simulink model "TopLevelSim"  (R2024b)
settings: Solver=FixedStepDiscrete  StartTime=0.0  StopTime=sysParams.FPGAClkPeriod*1e4  RelTol=1e-3
PreLoadFcn:
  | init;
undefined symbols (not defined in the file): bfCoeffs_fxp, chanConfig, const_16APSK, const_64APSK, FXP, iChain, modEnable, modSel, OFDMmodType, SC, SCmodType, sysParams, tuningWord, txData
libraries: hdlsllib x20, commdigbbndpm3 x8, commdigbbndam3 x8, dspmlti4 x8, dsphdlfiltering2 x8, whdlmod x4, dsphdlsigops2 x4
(part 2 of 2)

== system TopLevelSim/Top Level/Baseband Signal Generator/channel1/Baseband Modulator/OFDM Modulator/mapper ==
  txBits : Inport
  OFDMmodType : Inport  Port=2
  16-APSK : LookupNDDirect  NumberOfTableDimensions=1  Table=const_16APSK  DiagnosticForOutOfRangeInput=Error
  64-APSK : LookupNDDirect  NumberOfTableDimensions=1  Table=const_64APSK  DiagnosticForOutOfRangeInput=Error
  Bit Slice : hdlsllib/Logic and Bit Operations/Bit Slice  lidx=3  ridx=0
  Bit Slice1 : hdlsllib/Logic and Bit Operations/Bit Slice  lidx=1  ridx=0
  Multiport Switch : MultiPortSwitch  DataPortOrder=Zero-based contiguous  Inputs=4  zeroidx=on  OutDataTypeStr=fixdt(1,FXP.sampWL,FXP.sampFL)  SaturateOnIntegerOverflow=off
  QPSK Modulator Baseband : commdigbbndpm3/QPSK Modulator Baseband  InType=Integer  Enc=Gray  Ph=pi/4  outDtype=Fixed-point  outWordLen=FXP.sampWL  outUDDataType=sfix(16)  outFracLenMode=User-defined  outFracLen=FXP.sampFL  outDataTypeStr=fixdt(1,FXP.sampWL,FXP.sampFL)  outLastDataTypeStr=fixdt(1,FXP.sampWL,FXP.sampFL)
  Rectangular QAM Modulator Baseband : commdigbbndam3/Rectangular QAM Modulator Baseband  M=16  InType=Integer  Enc=Gray  Mapping=[0:15]  PowType=Average Power  MinDist=2  AvgPow=1  PeakPow=1  Ph=0  outDtype=Fixed-point  outWordLen=FXP.sampWL  outUDDataType=sfix(16)  outFracLenMode=User-defined  outFracLen=FXP.sampFL  outDataTypeStr=fixdt(1,FXP.sampWL,FXP.sampFL)  outLastDataTypeStr=fixdt(1,FXP.sampWL,FXP.sampFL)
  tx_IQ : Outport  VectorParamsAs1DForOutWhenUnconnected=off
  wires:
  Bit Slice1/1 -> QPSK Modulator Baseband/1
  Bit Slice/1 -> 16-APSK/1, Rectangular QAM Modulator Baseband/1
  txBits/1 -> Bit Slice1/1, Bit Slice/1, 64-APSK/1
  Multiport Switch/1 -> tx_IQ/1
  64-APSK/1 -> Multiport Switch/5
  16-APSK/1 -> Multiport Switch/4
  Rectangular QAM Modulator Baseband/1 -> Multiport Switch/3
  QPSK Modulator Baseband/1 -> Multiport Switch/2
  OFDMmodType/1 -> Multiport Switch/1

== system TopLevelSim/Top Level/Baseband Signal Generator/channel1/Baseband Modulator/SC Modulator/mapper ==
  txBits : Inport
  SCmodType : Inport  Port=2
  16-APSK : LookupNDDirect  NumberOfTableDimensions=1  Table=const_16APSK  DiagnosticForOutOfRangeInput=Error  TableDataTypeStr=fixdt(1,FXP.sampWL,FXP.sampFL)
  Bit Slice : hdlsllib/Logic and Bit Operations/Bit Slice  lidx=3  ridx=0
  Bit Slice1 : hdlsllib/Logic and Bit Operations/Bit Slice  lidx=1  ridx=0
  Multiport Switch : MultiPortSwitch  DataPortOrder=Zero-based contiguous  zeroidx=on  OutDataTypeStr=fixdt(1,FXP.sampWL,FXP.sampFL)  SaturateOnIntegerOverflow=off  InputSameDT=off
  QPSK Modulator Baseband : commdigbbndpm3/QPSK Modulator Baseband  InType=Integer  Enc=Gray  Ph=pi/4  outDtype=Fixed-point  outWordLen=FXP.sampWL  outUDDataType=sfix(16)  outFracLenMode=User-defined  outFracLen=FXP.sampFL  outDataTypeStr=fixdt(1,FXP.sampWL,FXP.sampFL)  outLastDataTypeStr=fixdt(1,FXP.sampWL,FXP.sampFL)
  Rectangular QAM Modulator Baseband : commdigbbndam3/Rectangular QAM Modulator Baseband  M=16  InType=Integer  Enc=Gray  Mapping=[0:15]  PowType=Average Power  MinDist=2  AvgPow=1  PeakPow=1  Ph=0  outDtype=Fixed-point  outWordLen=FXP.sampWL  outUDDataType=sfix(16)  outFracLenMode=User-defined  outFracLen=FXP.sampFL  outDataTypeStr=fixdt(1,FXP.sampWL,FXP.sampFL)  outLastDataTypeStr=fixdt(1,FXP.sampWL,FXP.sampFL)
  tx_IQ : Outport
  wires:
  Bit Slice1/1 -> QPSK Modulator Baseband/1
  Bit Slice/1 -> 16-APSK/1, Rectangular QAM Modulator Baseband/1
  txBits/1 -> Bit Slice1/1, Bit Slice/1
  QPSK Modulator Baseband/1 -> Multiport Switch/2
  Rectangular QAM Modulator Baseband/1 -> Multiport Switch/4
  SCmodType/1 -> Multiport Switch/1
  Multiport Switch/1 -> tx_IQ/1
  16-APSK/1 -> Multiport Switch/3

== system TopLevelSim/Top Level/Baseband Signal Generator/channel2/Baseband Modulator/OFDM Modulator/mapper ==
  txBits : Inport
  OFDMmodType : Inport  Port=2
  16-APSK : LookupNDDirect  NumberOfTableDimensions=1  Table=const_16APSK  DiagnosticForOutOfRangeInput=Error
  64-APSK : LookupNDDirect  NumberOfTableDimensions=1  Table=const_64APSK  DiagnosticForOutOfRangeInput=Error
  Bit Slice : hdlsllib/Logic and Bit Operations/Bit Slice  lidx=3  ridx=0
  Bit Slice1 : hdlsllib/Logic and Bit Operations/Bit Slice  lidx=1  ridx=0
  Multiport Switch : MultiPortSwitch  DataPortOrder=Zero-based contiguous  Inputs=4  zeroidx=on  OutDataTypeStr=fixdt(1,FXP.sampWL,FXP.sampFL)  SaturateOnIntegerOverflow=off
  QPSK Modulator Baseband : commdigbbndpm3/QPSK Modulator Baseband  InType=Integer  Enc=Gray  Ph=pi/4  outDtype=Fixed-point  outWordLen=FXP.sampWL  outUDDataType=sfix(16)  outFracLenMode=User-defined  outFracLen=FXP.sampFL  outDataTypeStr=fixdt(1,FXP.sampWL,FXP.sampFL)  outLastDataTypeStr=fixdt(1,FXP.sampWL,FXP.sampFL)
  Rectangular QAM Modulator Baseband : commdigbbndam3/Rectangular QAM Modulator Baseband  M=16  InType=Integer  Enc=Gray  Mapping=[0:15]  PowType=Average Power  MinDist=2  AvgPow=1  PeakPow=1  Ph=0  outDtype=Fixed-point  outWordLen=FXP.sampWL  outUDDataType=sfix(16)  outFracLenMode=User-defined  outFracLen=FXP.sampFL  outDataTypeStr=fixdt(1,FXP.sampWL,FXP.sampFL)  outLastDataTypeStr=fixdt(1,FXP.sampWL,FXP.sampFL)
  tx_IQ : Outport  VectorParamsAs1DForOutWhenUnconnected=off
  wires:
  OFDMmodType/1 -> Multiport Switch/1
  QPSK Modulator Baseband/1 -> Multiport Switch/2
  Rectangular QAM Modulator Baseband/1 -> Multiport Switch/3
  16-APSK/1 -> Multiport Switch/4
  64-APSK/1 -> Multiport Switch/5
  Multiport Switch/1 -> tx_IQ/1
  txBits/1 -> 64-APSK/1, Bit Slice/1, Bit Slice1/1
  Bit Slice/1 -> Rectangular QAM Modulator Baseband/1, 16-APSK/1
  Bit Slice1/1 -> QPSK Modulator Baseband/1

== system TopLevelSim/Top Level/Baseband Signal Generator/channel2/Baseband Modulator/SC Modulator/mapper ==
  txBits : Inport
  SCmodType : Inport  Port=2
  16-APSK : LookupNDDirect  NumberOfTableDimensions=1  Table=const_16APSK  DiagnosticForOutOfRangeInput=Error  TableDataTypeStr=fixdt(1,FXP.sampWL,FXP.sampFL)
  Bit Slice : hdlsllib/Logic and Bit Operations/Bit Slice  lidx=3  ridx=0
  Bit Slice1 : hdlsllib/Logic and Bit Operations/Bit Slice  lidx=1  ridx=0
  Multiport Switch : MultiPortSwitch  DataPortOrder=Zero-based contiguous  zeroidx=on  OutDataTypeStr=fixdt(1,FXP.sampWL,FXP.sampFL)  SaturateOnIntegerOverflow=off  InputSameDT=off
  QPSK Modulator Baseband : commdigbbndpm3/QPSK Modulator Baseband  InType=Integer  Enc=Gray  Ph=pi/4  outDtype=Fixed-point  outWordLen=FXP.sampWL  outUDDataType=sfix(16)  outFracLenMode=User-defined  outFracLen=FXP.sampFL  outDataTypeStr=fixdt(1,FXP.sampWL,FXP.sampFL)  outLastDataTypeStr=fixdt(1,FXP.sampWL,FXP.sampFL)
  Rectangular QAM Modulator Baseband : commdigbbndam3/Rectangular QAM Modulator Baseband  M=16  InType=Integer  Enc=Gray  Mapping=[0:15]  PowType=Average Power  MinDist=2  AvgPow=1  PeakPow=1  Ph=0  outDtype=Fixed-point  outWordLen=FXP.sampWL  outUDDataType=sfix(16)  outFracLenMode=User-defined  outFracLen=FXP.sampFL  outDataTypeStr=fixdt(1,FXP.sampWL,FXP.sampFL)  outLastDataTypeStr=fixdt(1,FXP.sampWL,FXP.sampFL)
  tx_IQ : Outport
  wires:
  16-APSK/1 -> Multiport Switch/3
  Multiport Switch/1 -> tx_IQ/1
  SCmodType/1 -> Multiport Switch/1
  Rectangular QAM Modulator Baseband/1 -> Multiport Switch/4
  QPSK Modulator Baseband/1 -> Multiport Switch/2
  txBits/1 -> Bit Slice/1, Bit Slice1/1
  Bit Slice/1 -> Rectangular QAM Modulator Baseband/1, 16-APSK/1
  Bit Slice1/1 -> QPSK Modulator Baseband/1

== system TopLevelSim/Top Level/Baseband Signal Generator/channel3/Baseband Modulator/OFDM Modulator/mapper ==
  txBits : Inport
  OFDMmodType : Inport  Port=2
  16-APSK : LookupNDDirect  NumberOfTableDimensions=1  Table=const_16APSK  DiagnosticForOutOfRangeInput=Error
  64-APSK : LookupNDDirect  NumberOfTableDimensions=1  Table=const_64APSK  DiagnosticForOutOfRangeInput=Error
  Bit Slice : hdlsllib/Logic and Bit Operations/Bit Slice  lidx=3  ridx=0
  Bit Slice1 : hdlsllib/Logic and Bit Operations/Bit Slice  lidx=1  ridx=0
  Multiport Switch : MultiPortSwitch  DataPortOrder=Zero-based contiguous  Inputs=4  zeroidx=on  OutDataTypeStr=fixdt(1,FXP.sampWL,FXP.sampFL)  SaturateOnIntegerOverflow=off
  QPSK Modulator Baseband : commdigbbndpm3/QPSK Modulator Baseband  InType=Integer  Enc=Gray  Ph=pi/4  outDtype=Fixed-point  outWordLen=FXP.sampWL  outUDDataType=sfix(16)  outFracLenMode=User-defined  outFracLen=FXP.sampFL  outDataTypeStr=fixdt(1,FXP.sampWL,FXP.sampFL)  outLastDataTypeStr=fixdt(1,FXP.sampWL,FXP.sampFL)
  Rectangular QAM Modulator Baseband : commdigbbndam3/Rectangular QAM Modulator Baseband  M=16  InType=Integer  Enc=Gray  Mapping=[0:15]  PowType=Average Power  MinDist=2  AvgPow=1  PeakPow=1  Ph=0  outDtype=Fixed-point  outWordLen=FXP.sampWL  outUDDataType=sfix(16)  outFracLenMode=User-defined  outFracLen=FXP.sampFL  outDataTypeStr=fixdt(1,FXP.sampWL,FXP.sampFL)  outLastDataTypeStr=fixdt(1,FXP.sampWL,FXP.sampFL)
  tx_IQ : Outport  VectorParamsAs1DForOutWhenUnconnected=off
  wires:
  Bit Slice1/1 -> QPSK Modulator Baseband/1
  Bit Slice/1 -> 16-APSK/1, Rectangular QAM Modulator Baseband/1
  txBits/1 -> Bit Slice1/1, Bit Slice/1, 64-APSK/1
  Multiport Switch/1 -> tx_IQ/1
  64-APSK/1 -> Multiport Switch/5
  16-APSK/1 -> Multiport Switch/4
  Rectangular QAM Modulator Baseband/1 -> Multiport Switch/3
  QPSK Modulator Baseband/1 -> Multiport Switch/2
  OFDMmodType/1 -> Multiport Switch/1

== system TopLevelSim/Top Level/Baseband Signal Generator/channel3/Baseband Modulator/SC Modulator/mapper ==
  txBits : Inport
  SCmodType : Inport  Port=2
  16-APSK : LookupNDDirect  NumberOfTableDimensions=1  Table=const_16APSK  DiagnosticForOutOfRangeInput=Error  TableDataTypeStr=fixdt(1,FXP.sampWL,FXP.sampFL)
  Bit Slice : hdlsllib/Logic and Bit Operations/Bit Slice  lidx=3  ridx=0
  Bit Slice1 : hdlsllib/Logic and Bit Operations/Bit Slice  lidx=1  ridx=0
  Multiport Switch : MultiPortSwitch  DataPortOrder=Zero-based contiguous  zeroidx=on  OutDataTypeStr=fixdt(1,FXP.sampWL,FXP.sampFL)  SaturateOnIntegerOverflow=off  InputSameDT=off
  QPSK Modulator Baseband : commdigbbndpm3/QPSK Modulator Baseband  InType=Integer  Enc=Gray  Ph=pi/4  outDtype=Fixed-point  outWordLen=FXP.sampWL  outUDDataType=sfix(16)  outFracLenMode=User-defined  outFracLen=FXP.sampFL  outDataTypeStr=fixdt(1,FXP.sampWL,FXP.sampFL)  outLastDataTypeStr=fixdt(1,FXP.sampWL,FXP.sampFL)
  Rectangular QAM Modulator Baseband : commdigbbndam3/Rectangular QAM Modulator Baseband  M=16  InType=Integer  Enc=Gray  Mapping=[0:15]  PowType=Average Power  MinDist=2  AvgPow=1  PeakPow=1  Ph=0  outDtype=Fixed-point  outWordLen=FXP.sampWL  outUDDataType=sfix(16)  outFracLenMode=User-defined  outFracLen=FXP.sampFL  outDataTypeStr=fixdt(1,FXP.sampWL,FXP.sampFL)  outLastDataTypeStr=fixdt(1,FXP.sampWL,FXP.sampFL)
  tx_IQ : Outport
  wires:
  Bit Slice1/1 -> QPSK Modulator Baseband/1
  Bit Slice/1 -> 16-APSK/1, Rectangular QAM Modulator Baseband/1
  txBits/1 -> Bit Slice1/1, Bit Slice/1
  QPSK Modulator Baseband/1 -> Multiport Switch/2
  Rectangular QAM Modulator Baseband/1 -> Multiport Switch/4
  SCmodType/1 -> Multiport Switch/1
  Multiport Switch/1 -> tx_IQ/1
  16-APSK/1 -> Multiport Switch/3

== system TopLevelSim/Top Level/Baseband Signal Generator/channel4/Baseband Modulator/OFDM Modulator/mapper ==
  txBits : Inport
  OFDMmodType : Inport  Port=2
  16-APSK : LookupNDDirect  NumberOfTableDimensions=1  Table=const_16APSK  DiagnosticForOutOfRangeInput=Error
  64-APSK : LookupNDDirect  NumberOfTableDimensions=1  Table=const_64APSK  DiagnosticForOutOfRangeInput=Error
  Bit Slice : hdlsllib/Logic and Bit Operations/Bit Slice  lidx=3  ridx=0
  Bit Slice1 : hdlsllib/Logic and Bit Operations/Bit Slice  lidx=1  ridx=0
  Multiport Switch : MultiPortSwitch  DataPortOrder=Zero-based contiguous  Inputs=4  zeroidx=on  OutDataTypeStr=fixdt(1,FXP.sampWL,FXP.sampFL)  SaturateOnIntegerOverflow=off
  QPSK Modulator Baseband : commdigbbndpm3/QPSK Modulator Baseband  InType=Integer  Enc=Gray  Ph=pi/4  outDtype=Fixed-point  outWordLen=FXP.sampWL  outUDDataType=sfix(16)  outFracLenMode=User-defined  outFracLen=FXP.sampFL  outDataTypeStr=fixdt(1,FXP.sampWL,FXP.sampFL)  outLastDataTypeStr=fixdt(1,FXP.sampWL,FXP.sampFL)
  Rectangular QAM Modulator Baseband : commdigbbndam3/Rectangular QAM Modulator Baseband  M=16  InType=Integer  Enc=Gray  Mapping=[0:15]  PowType=Average Power  MinDist=2  AvgPow=1  PeakPow=1  Ph=0  outDtype=Fixed-point  outWordLen=FXP.sampWL  outUDDataType=sfix(16)  outFracLenMode=User-defined  outFracLen=FXP.sampFL  outDataTypeStr=fixdt(1,FXP.sampWL,FXP.sampFL)  outLastDataTypeStr=fixdt(1,FXP.sampWL,FXP.sampFL)
  tx_IQ : Outport  VectorParamsAs1DForOutWhenUnconnected=off
  wires:
  OFDMmodType/1 -> Multiport Switch/1
  QPSK Modulator Baseband/1 -> Multiport Switch/2
  Rectangular QAM Modulator Baseband/1 -> Multiport Switch/3
  16-APSK/1 -> Multiport Switch/4
  64-APSK/1 -> Multiport Switch/5
  Multiport Switch/1 -> tx_IQ/1
  txBits/1 -> 64-APSK/1, Bit Slice/1, Bit Slice1/1
  Bit Slice/1 -> Rectangular QAM Modulator Baseband/1, 16-APSK/1
  Bit Slice1/1 -> QPSK Modulator Baseband/1

== system TopLevelSim/Top Level/Baseband Signal Generator/channel4/Baseband Modulator/SC Modulator/mapper ==
  txBits : Inport
  SCmodType : Inport  Port=2
  16-APSK : LookupNDDirect  NumberOfTableDimensions=1  Table=const_16APSK  DiagnosticForOutOfRangeInput=Error  TableDataTypeStr=fixdt(1,FXP.sampWL,FXP.sampFL)
  Bit Slice : hdlsllib/Logic and Bit Operations/Bit Slice  lidx=3  ridx=0
  Bit Slice1 : hdlsllib/Logic and Bit Operations/Bit Slice  lidx=1  ridx=0
  Multiport Switch : MultiPortSwitch  DataPortOrder=Zero-based contiguous  zeroidx=on  OutDataTypeStr=fixdt(1,FXP.sampWL,FXP.sampFL)  SaturateOnIntegerOverflow=off  InputSameDT=off
  QPSK Modulator Baseband : commdigbbndpm3/QPSK Modulator Baseband  InType=Integer  Enc=Gray  Ph=pi/4  outDtype=Fixed-point  outWordLen=FXP.sampWL  outUDDataType=sfix(16)  outFracLenMode=User-defined  outFracLen=FXP.sampFL  outDataTypeStr=fixdt(1,FXP.sampWL,FXP.sampFL)  outLastDataTypeStr=fixdt(1,FXP.sampWL,FXP.sampFL)
  Rectangular QAM Modulator Baseband : commdigbbndam3/Rectangular QAM Modulator Baseband  M=16  InType=Integer  Enc=Gray  Mapping=[0:15]  PowType=Average Power  MinDist=2  AvgPow=1  PeakPow=1  Ph=0  outDtype=Fixed-point  outWordLen=FXP.sampWL  outUDDataType=sfix(16)  outFracLenMode=User-defined  outFracLen=FXP.sampFL  outDataTypeStr=fixdt(1,FXP.sampWL,FXP.sampFL)  outLastDataTypeStr=fixdt(1,FXP.sampWL,FXP.sampFL)
  tx_IQ : Outport
  wires:
  16-APSK/1 -> Multiport Switch/3
  Multiport Switch/1 -> tx_IQ/1
  SCmodType/1 -> Multiport Switch/1
  Rectangular QAM Modulator Baseband/1 -> Multiport Switch/4
  QPSK Modulator Baseband/1 -> Multiport Switch/2
  txBits/1 -> Bit Slice/1, Bit Slice1/1
  Bit Slice/1 -> Rectangular QAM Modulator Baseband/1, 16-APSK/1
  Bit Slice1/1 -> QPSK Modulator Baseband/1
